simulink library "suspension_lib"  (Simulink 7.6)
settings: Solver=ode45  StartTime=0.0  StopTime=10.0  RelTol=1e-3
libraries: suspension_lib x2
settings Model: Creator=heminggs  LastModifiedBy=heminggs

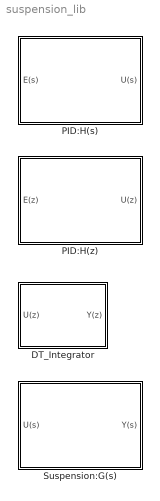
== system suspension_lib ==
  DT_Integrator : Subsystem  mask{Ts=.01, X0=0, X_MIN=-inf, X_MAX=inf}
      mask prompts: Ts "Ts (seconds)"
  PID:H(s) : Subsystem  mask{K_P=200000, K_D=100, tau_D=.01/pi, P_MAX=1500*2, P_MIN=-1500*2, X_DMAX=1500*2, X_DMIN=-1500*2, X_D0=0, K_I=600000, X_IMAX=1500, X_IMIN=-1500, X_I0=0}
  PID:H(z) : Subsystem  mask{Ts=.01, K_P=200000, K_D=100, tau_D=.01/pi, P_MAX=1500*2, P_MIN=-1500*2, X_DMAX=1500*2, X_DMIN=-1500*2, X_D0=0, K_I=600000, X_IMAX=1500, X_IMIN=-1500, X_I0=0}
      mask prompts: Ts "Ts (seconds)"
  Suspension:G(s) : Subsystem  mask{k=31000, m=15, c=830, U_MAX=1500}
      mask prompts: k "k (N/m)"; m "m (kg)"; c "c (N-s/m)"; U_MAX "u_max (N)"
      mask init:
      | omega_n=sqrt(k/m);
      | zet=c/(2*sqrt(k*m));

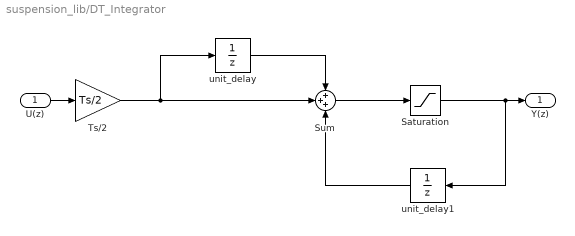
== system suspension_lib/DT_Integrator ==
  U(z) : Inport
  Saturation : Saturate  UpperLimit=X_MAX  LowerLimit=X_MIN
  Sum : Sum  Inputs=+++
  Ts/2 : Gain  Gain=Ts/2
  unit_delay : UnitDelay  SampleTime=Ts
  unit_delay1 : UnitDelay  X0=X0  SampleTime=Ts
  Y(z) : Outport
  wires:
  U(z)/1 -> Ts/2/1
  Ts/2/1 -> Sum/2, unit_delay/1
  unit_delay1/1 -> Sum/3
  Saturation/1 -> Y(z)/1, unit_delay1/1
  Sum/1 -> Saturation/1
  unit_delay/1 -> Sum/1

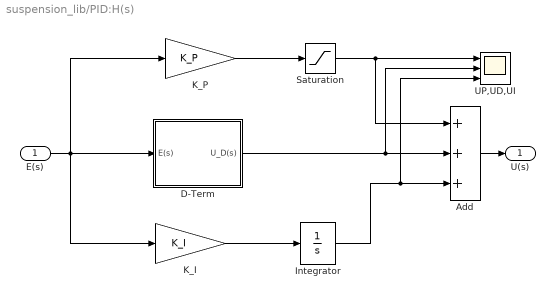
== system suspension_lib/PID:H(s) ==
  E(s) : Inport
  Add : Sum  Inputs=+++
  D-Term : Subsystem
  Integrator : Integrator  InitialCondition=X_I0  LimitOutput=on  UpperSaturationLimit=X_IMAX  LowerSaturationLimit=X_IMIN
  K_I : Gain  Gain=K_I
  K_P : Gain  Gain=K_P
  Saturation : Saturate  UpperLimit=P_MAX  LowerLimit=P_MIN
  UP,UD,UI : Scope  NumInputPorts=3
      settings: YMin=-5~-5~-5  YMax=5~5~5
  U(s) : Outport
  wires:
  Add/1 -> U(s)/1
  D-Term/1(U_D(s)) -> Add/2, UP,UD,UI/2
  Integrator/1 -> Add/3, UP,UD,UI/3
  K_I/1 -> Integrator/1
  K_P/1 -> Saturation/1
  E(s)/1 -> D-Term/1(E(s)), K_I/1, K_P/1
  Saturation/1 -> Add/1, UP,UD,UI/1

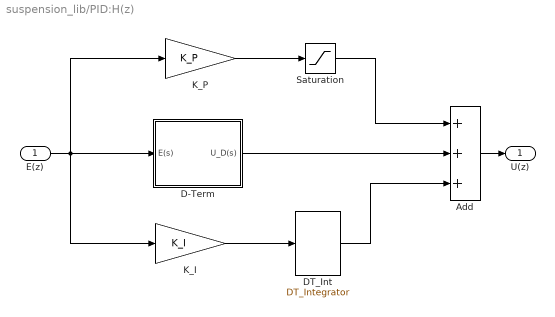
== system suspension_lib/PID:H(z) ==
  E(z) : Inport
  Add : Sum  Inputs=+++
  D-Term : Subsystem
  DT_Int : suspension_lib/DT_Integrator  SystemSampleTime=-1  Ts=Ts  X0=X_I0  X_MIN=X_IMIN  X_MAX=X_IMAX
  K_I : Gain  Gain=K_I
  K_P : Gain  Gain=K_P
  Saturation : Saturate  UpperLimit=P_MAX  LowerLimit=P_MIN
  U(z) : Outport
  wires:
  E(z)/1 -> K_P/1, K_I/1, D-Term/1(E(s))
  K_P/1 -> Saturation/1
  K_I/1 -> DT_Int/1
  DT_Int/1 -> Add/3
  D-Term/1(U_D(s)) -> Add/2
  Add/1 -> U(z)/1
  Saturation/1 -> Add/1

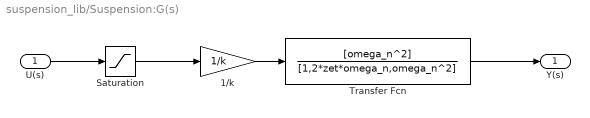
== system suspension_lib/Suspension:G(s) ==
  U(s) : Inport
  1/k : Gain  Gain=1/k
  Saturation : Saturate  UpperLimit=U_MAX  LowerLimit=-U_MAX
  Transfer Fcn : TransferFcn  Numerator=[omega_n^2]  Denominator=[1,2*zet*omega_n,omega_n^2]
  Y(s) : Outport
  wires:
  Transfer Fcn/1 -> Y(s)/1
  1/k/1 -> Transfer Fcn/1
  Saturation/1 -> 1/k/1
  U(s)/1 -> Saturation/1

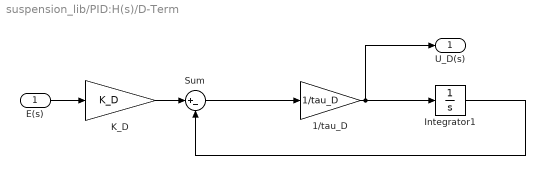
== system suspension_lib/PID:H(s)/D-Term ==
  E(s) : Inport
  1/tau_D : Gain  Gain=1/tau_D
  Integrator1 : Integrator  InitialCondition=X_D0  LimitOutput=on  UpperSaturationLimit=X_DMAX*tau_D  LowerSaturationLimit=X_DMIN*tau_D
  K_D : Gain  Gain=K_D
  Sum : Sum  Inputs=|+-
  U_D(s) : Outport
  wires:
  E(s)/1 -> K_D/1
  1/tau_D/1 -> U_D(s)/1, Integrator1/1
  Integrator1/1 -> Sum/2
  K_D/1 -> Sum/1
  Sum/1 -> 1/tau_D/1

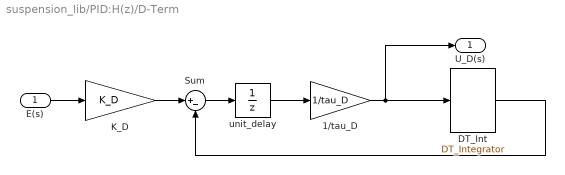
== system suspension_lib/PID:H(z)/D-Term ==
  E(s) : Inport
  1/tau_D : Gain  Gain=1/tau_D
  DT_Int : suspension_lib/DT_Integrator  SystemSampleTime=-1  Ts=Ts  X0=X_D0  X_MIN=X_DMIN*tau_D  X_MAX=X_DMAX*tau_D
  K_D : Gain  Gain=K_D
  Sum : Sum  Inputs=|+-
  unit_delay : UnitDelay  SampleTime=Ts
  U_D(s) : Outport
  wires:
  K_D/1 -> Sum/1
  DT_Int/1 -> Sum/2
  1/tau_D/1 -> DT_Int/1, U_D(s)/1
  E(s)/1 -> K_D/1
  Sum/1 -> unit_delay/1
  unit_delay/1 -> 1/tau_D/1
